simulink library "uavsimBlockset_AirspeedController"  (Simulink 8.0)
settings: Solver=ode45  StartTime=0.0  StopTime=10.0  RelTol=1e-3
settings Model: Creator=mstolle  LastModifiedBy=j.bolting

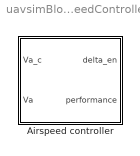
== system uavsimBlockset_AirspeedController ==
  Airspeed controller : Subsystem  mask{mask_K=0}
      mask prompts: mask_K "Feedback gain matrix K"

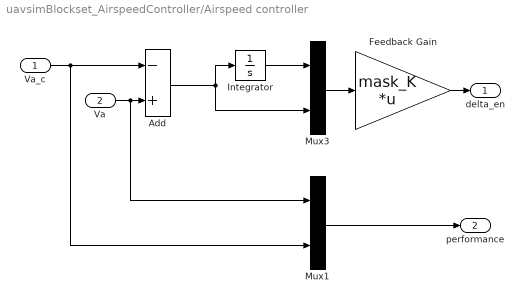
== system uavsimBlockset_AirspeedController/Airspeed controller ==
  Va_c : Inport
  Va : Inport  Port=2
  Add : Sum  Inputs=-+
  Feedback Gain : Gain  Gain=mask_K  Multiplication=Matrix(K*u)
  Integrator : Integrator
  Mux1 : Mux  Inputs=2
  Mux3 : Mux  Inputs=2
  delta_en : Outport
  performance : Outport  Port=2
  wires:
  Integrator/1 -> Mux3/1
  Va_c/1 -> Mux1/2, Add/1
  Add/1 -> Integrator/1, Mux3/2
  Mux3/1 -> Feedback Gain/1
  Feedback Gain/1 -> delta_en/1
  Mux1/1 -> performance/1
  Va/1 -> Mux1/1, Add/2
